simulink model "pd_plus_testings_7DOF_alternative"  (R2022b)
settings: Solver=ode4  StartTime=0.0  StopTime=101  FixedStep=1e-3  RelTol=1e-3
InitFcn:
  | parameters_7dof;
undefined symbols (not defined in the file): param_robot, q_0
(part 1 of 7)
settings Model: Creator=emu  LastModifiedBy=emu

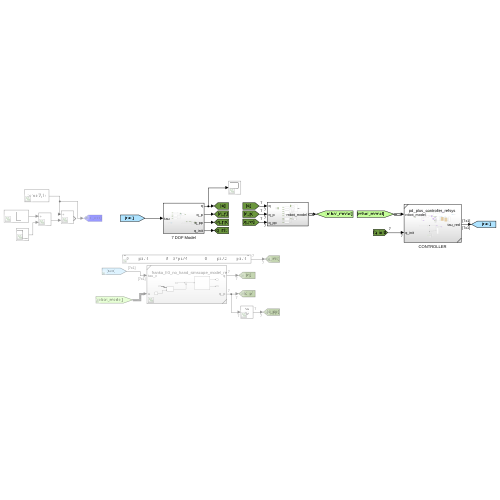
[thumbnail: Simulink's stored preview of the top-level diagram]
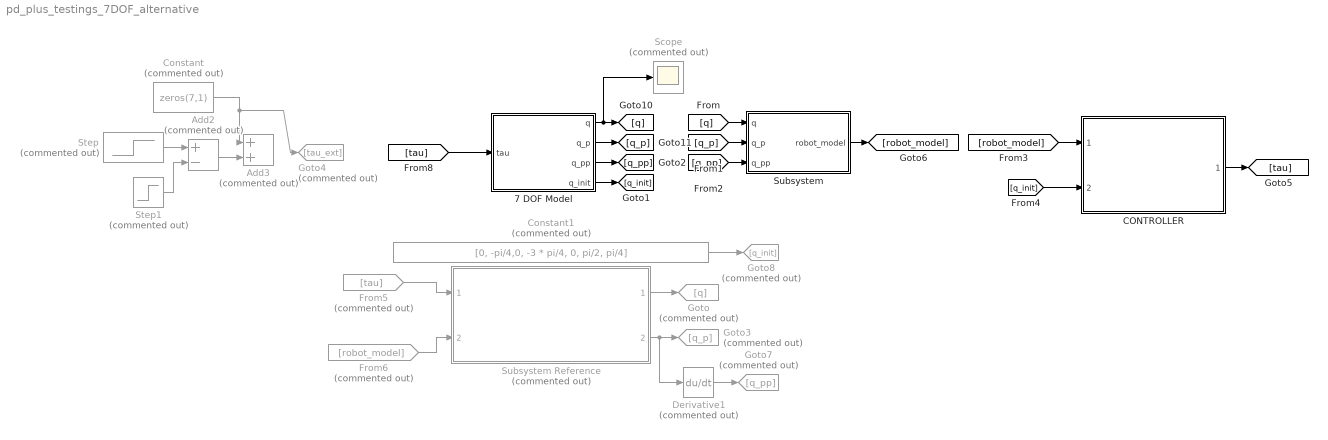
== system pd_plus_testings_7DOF_alternative ==
  7 DOF Model : Subsystem
  Add2 : Sum  Commented=on  Inputs=+-
  Add3 : Sum  Commented=on
  CONTROLLER : Subsystem  ReferencedSubsystem=pd_plus_controller_refsys
  Constant : Constant  Commented=on  Value=zeros(7,1)
  Constant1 : Constant  Commented=on  Value=[0, -pi/4,0, -3 * pi/4, 0, pi/2, pi/4]
  Derivative1 : Derivative  Commented=on
  From5 : From  Commented=on  GotoTag=tau
  From6 : From  Commented=on  GotoTag=robot_model
  Goto : Goto  Commented=on  GotoTag=q
  Goto3 : Goto  Commented=on  GotoTag=q_p
  Goto4 : Goto  Commented=on  GotoTag=tau_ext
  Goto7 : Goto  Commented=on  GotoTag=q_pp
  Goto8 : Goto  Commented=on  GotoTag=q_init
  Scope : Scope  Commented=on
  Step : Step  Commented=on  Time=2  Before=1  After=0  SampleTime=0
  Step1 : Step  Commented=on  Before=1  After=0  SampleTime=0
  Subsystem : Subsystem
  Subsystem Reference : Subsystem  Commented=on  ReferencedSubsystem=franka_fr3_no_hand_simscape_model_refsys
  wires:
  [q] -> Subsystem/1(q)
  [q_pp] -> Subsystem/3(q_pp)
  [q_p] -> Subsystem/2(q_p)
  [robot_model] -> CONTROLLER/1
  Step/1 -> Add2/1
  Step1/1 -> Add2/2
  Add2/1 -> Add3/2
  7 DOF Model/1(q) -> Scope/1, [q]
  7 DOF Model/2(q_p) -> [q_p]
  7 DOF Model/3(q_pp) -> [q_pp]
  [tau] -> 7 DOF Model/1(tau)
  Subsystem/1(robot_model) -> [robot_model]
  CONTROLLER/1 -> [tau]
  Constant/1 -> Goto4/1, Add3/1
  7 DOF Model/4(q_init) -> [q_init]
  [q_init] -> CONTROLLER/2
  From5/1 -> Subsystem Reference/1
  Subsystem Reference/1 -> Goto/1
  Subsystem Reference/2 -> Derivative1/1, Goto3/1
  Derivative1/1 -> Goto7/1
  Constant1/1 -> Goto8/1
  From6/1 -> Subsystem Reference/2

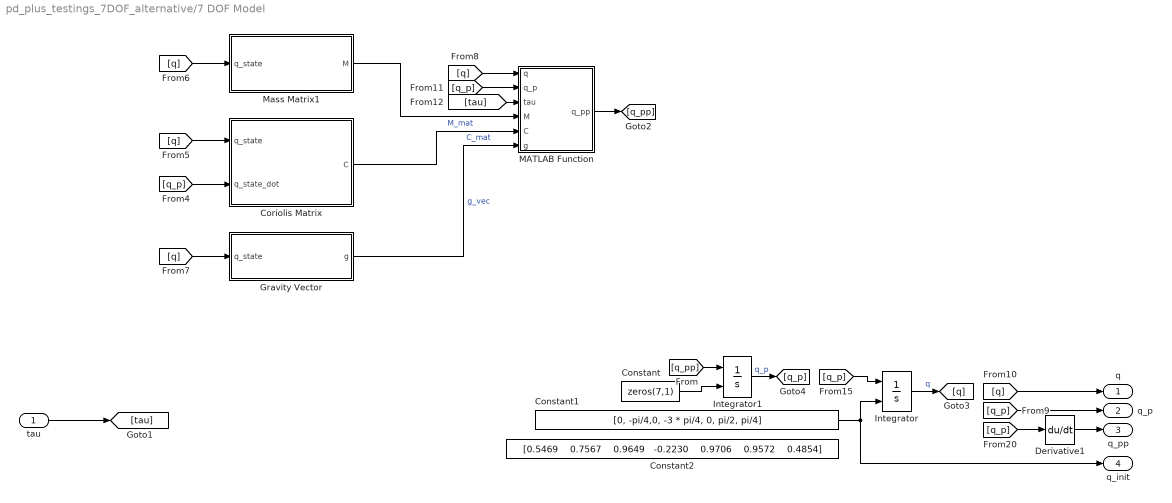
== system pd_plus_testings_7DOF_alternative/7 DOF Model ==
  tau : Inport
  Constant : Constant  Value=zeros(7,1)
  Constant1 : Constant  Value=[0, -pi/4,0, -3 * pi/4, 0, pi/2, pi/4]
  Constant2 : Constant  Value="[0.5469    0.7567    0.9649   -0.2230    0.9706    0.9572    0.4854]"
  Coriolis Matrix : MATLAB Function  TreatAsAtomicUnit=on
  Derivative1 : Derivative
  Gravity Vector : MATLAB Function  TreatAsAtomicUnit=on
  Integrator : Integrator  InitialConditionSource=external  InitialCondition=q_0  UpperSaturationLimit=param_robot.q_limit_upper  LowerSaturationLimit=param_robot.q_limit_lower
  Integrator1 : Integrator  InitialConditionSource=external  InitialCondition=param_robot.q_0_p_ref  UpperSaturationLimit=param_robot.q_p_limit_upper  LowerSaturationLimit=param_robot.q_p_limit_lower
  MATLAB Function : MATLAB Function  TreatAsAtomicUnit=on
  Mass Matrix1 : MATLAB Function  TreatAsAtomicUnit=on
  q : Outport
  q_p : Outport  Port=2
  q_pp : Outport  Port=3
  q_init : Outport  Port=4
  wires:
  [q_p] -> Derivative1/1
  Derivative1/1 -> q_pp/1
  tau/1 -> [tau]
  [q_p] -> q_p/1
  [q_p] -> Integrator/1
  Integrator1/1 -> [q_p]  "q_p"
  Integrator/1 -> [q]  "q"
  [q] -> q/1
  [q_pp] -> Integrator1/1
  Constant/1 -> Integrator1/2
  Constant1/1 -> q_init/1, Integrator/2
  [q_p] -> Coriolis Matrix/2(q_state_dot)
  [q] -> Coriolis Matrix/1(q_state)
  [q] -> Mass Matrix1/1(q_state)
  [q] -> Gravity Vector/1(q_state)
  Mass Matrix1/1(M) -> MATLAB Function/4(M)  "M_mat"
  Coriolis Matrix/1(C) -> MATLAB Function/5(C)  "C_mat"
  Gravity Vector/1(g) -> MATLAB Function/6(g)  "g_vec"
  [q] -> MATLAB Function/1(q)
  [q_p] -> MATLAB Function/2(q_p)
  [tau] -> MATLAB Function/3(tau)
  MATLAB Function/1(q_pp) -> [q_pp]

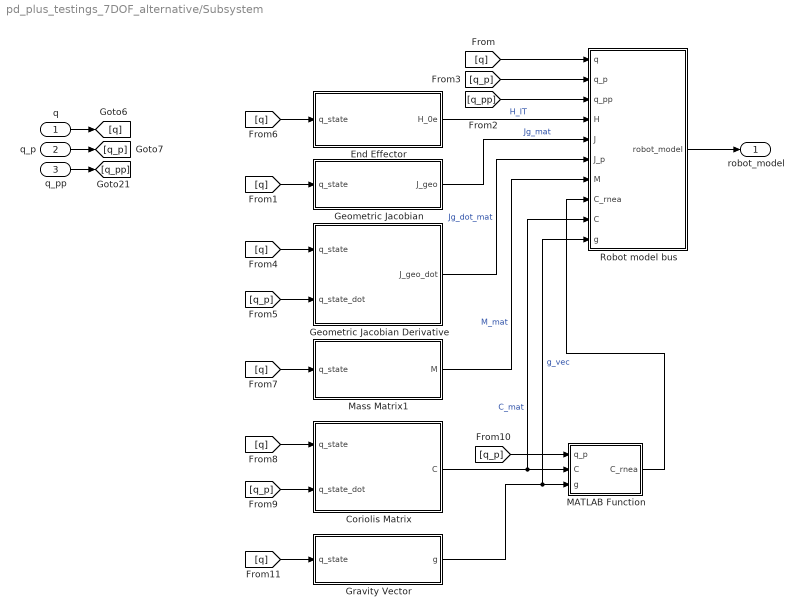
== system pd_plus_testings_7DOF_alternative/Subsystem ==
  q : Inport
  q_p : Inport  Port=2
  q_pp : Inport  Port=3
  Coriolis Matrix : MATLAB Function  TreatAsAtomicUnit=on
  End Effector : MATLAB Function  TreatAsAtomicUnit=on
  Geometric Jacobian : MATLAB Function  TreatAsAtomicUnit=on
  Geometric Jacobian Derivative : MATLAB Function  TreatAsAtomicUnit=on
  Gravity Vector : MATLAB Function  TreatAsAtomicUnit=on
  MATLAB Function : MATLAB Function  TreatAsAtomicUnit=on
  Mass Matrix1 : MATLAB Function  TreatAsAtomicUnit=on
  Robot model bus : MATLAB Function  TreatAsAtomicUnit=on
  robot_model : Outport  OutDataTypeStr=Bus: robot_model
  wires:
  q_pp/1 -> [q_pp]
  q_p/1 -> [q_p]
  q/1 -> [q]
  [q] -> End Effector/1(q_state)
  Robot model bus/1(robot_model) -> robot_model/1
  [q_pp] -> Robot model bus/3(q_pp)
  [q] -> Robot model bus/1(q)
  [q_p] -> Robot model bus/2(q_p)
  [q_p] -> Geometric Jacobian Derivative/2(q_state_dot)
  End Effector/1(H_0e) -> Robot model bus/4(H)  "H_IT"
  Geometric Jacobian/1(J_geo) -> Robot model bus/5(J)  "Jg_mat"
  [q] -> Geometric Jacobian/1(q_state)
  [q] -> Geometric Jacobian Derivative/1(q_state)
  Geometric Jacobian Derivative/1(J_geo_dot) -> Robot model bus/6(J_p)  "Jg_dot_mat"
  [q] -> Mass Matrix1/1(q_state)
  Mass Matrix1/1(M) -> Robot model bus/7(M)  "M_mat"
  [q] -> Coriolis Matrix/1(q_state)
  [q_p] -> Coriolis Matrix/2(q_state_dot)
  Coriolis Matrix/1(C) -> MATLAB Function/2(C), Robot model bus/9(C)  "C_mat"
  [q_p] -> MATLAB Function/1(q_p)
  [q] -> Gravity Vector/1(q_state)
  Gravity Vector/1(g) -> Robot model bus/10(g), MATLAB Function/3(g)  "g_vec"
  MATLAB Function/1(C_rnea) -> Robot model bus/8(C_rnea)
